simulink model "My_own_6dofblock"  (R2024b)
settings: Solver=VariableStepAuto  StartTime=0.0  StopTime=10.0  RelTol=1e-3
settings Model: Creator=Thetw  LastModifiedBy=Thetw

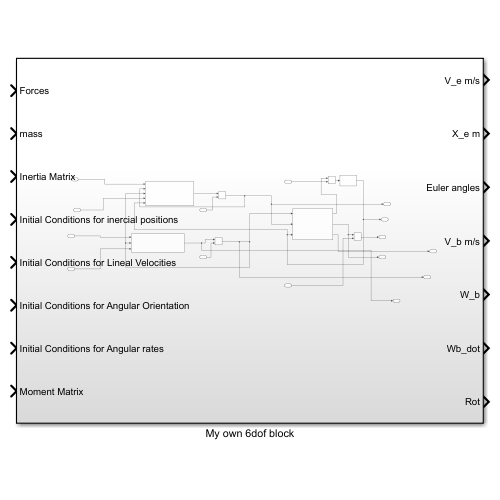
[thumbnail: Simulink's stored preview of the top-level diagram]
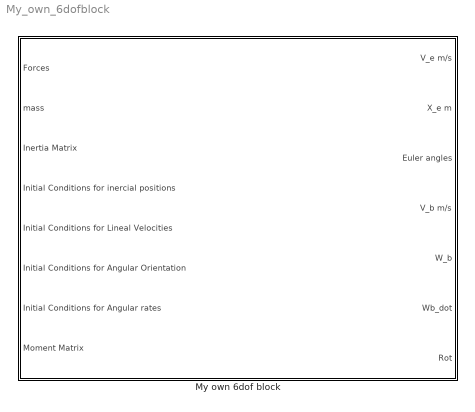
== system My_own_6dofblock ==
  My own 6dof block : Subsystem

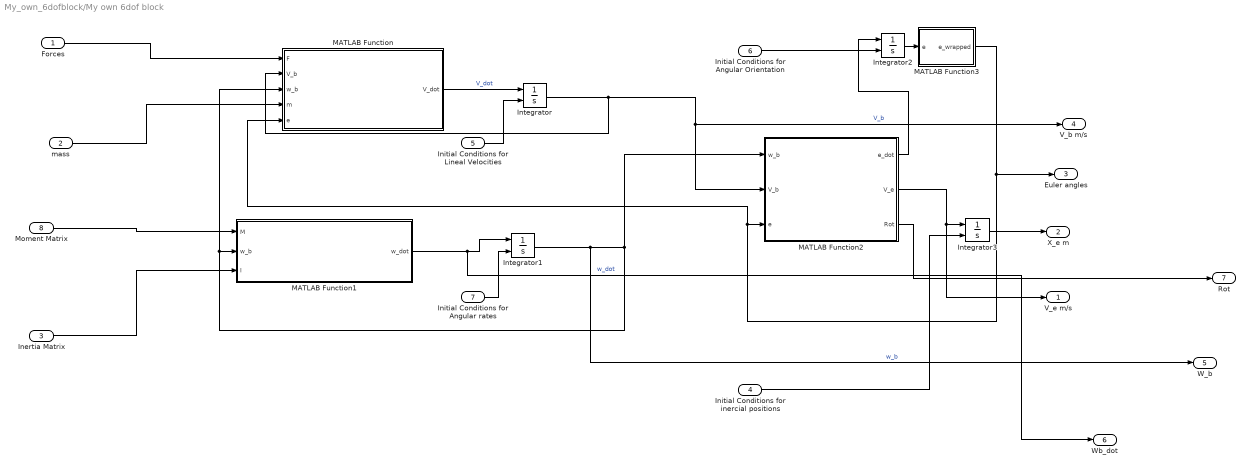
== system My_own_6dofblock/My own 6dof block ==
  Forces : Inport
  mass : Inport  Port=2
  Inertia Matrix : Inport  Port=3
  Initial Conditions for inercial positions : Inport  Port=4
  Initial Conditions for Lineal Velocities : Inport  Port=5
  Initial Conditions for Angular Orientation : Inport  Port=6
  Initial Conditions for Angular rates : Inport  Port=7
  Moment Matrix : Inport  Port=8
  Integrator{,1..3} (4 alike) : Integrator  InitialConditionSource=external
  MATLAB Function : MATLAB Function  TreatAsAtomicUnit=on
  MATLAB Function1 : MATLAB Function  TreatAsAtomicUnit=on
  MATLAB Function2 : MATLAB Function  TreatAsAtomicUnit=on
  MATLAB Function3 : MATLAB Function  TreatAsAtomicUnit=on
  V_e m/s : Outport
  X_e m : Outport  Port=2
  Euler angles : Outport  Port=3
  V_b m/s : Outport  Port=4
  W_b : Outport  Port=5
  Wb_dot : Outport  Port=6
  Rot : Outport  Port=7
  wires:
  Integrator1/1 -> W_b/1, MATLAB Function2/1(w_b), MATLAB Function/3(w_b), MATLAB Function1/2(w_b)  "w_b"
  MATLAB Function/1(V_dot) -> Integrator/1  "V_dot"
  Integrator2/1 -> MATLAB Function3/1(e)
  MATLAB Function2/2(V_e) -> V_e m/s/1, Integrator3/1
  mass/1 -> MATLAB Function/4(m)
  MATLAB Function2/1(e_dot) -> Integrator2/1
  MATLAB Function1/1(w_dot) -> Wb_dot/1, Integrator1/1  "w_dot"
  Integrator3/1 -> X_e m/1
  Integrator/1 -> MATLAB Function/2(V_b), V_b m/s/1, MATLAB Function2/2(V_b)  "V_b"
  Inertia Matrix/1 -> MATLAB Function1/3(I)
  Forces/1 -> MATLAB Function/1(F)
  Moment Matrix/1 -> MATLAB Function1/1(M)
  Initial Conditions for Lineal Velocities/1 -> Integrator/2
  Initial Conditions for Angular rates/1 -> Integrator1/2
  Initial Conditions for inercial positions/1 -> Integrator3/2
  MATLAB Function2/3(Rot) -> Rot/1
  Initial Conditions for Angular Orientation/1 -> Integrator2/2
  MATLAB Function3/1(e_wrapped) -> Euler angles/1, MATLAB Function/5(e), MATLAB Function2/3(e)

== matlab function My_own_6dofblock/My own 6dof block/MATLAB Function ==
  data: F input; V_dot output; V_b input; w_b input; m input; e input
 function V_dot = Traslational_Dynamics(F, V_b, w_b, m, e)

    % Force inputs into a column vector
    F   = F(:);
    V_b = V_b(:);
    w_b = w_b(:);

    % Coriolis effect 
    cross_term = cross(w_b, V_b);


    
    phi = e(1);
    theta = e(2);
    psi = e(3);

    % --- Rotation Matrix ---
    cpsi = cos(psi); spsi = sin(psi);
    cth = cos(theta); sth = sin(theta);
    cphi = cos(phi); sphi = sin(phi);

    R_eb = [ ...
        cth*cpsi,  sphi*sth*cpsi - cphi*spsi,  cphi*sth*cpsi + sphi*spsi;
        cth*spsi,  sphi*sth*spsi + cphi*cpsi,  cphi*sth*spsi - sphi*cpsi;
        -sth,       sphi*cth,                 cphi*cth ];

    Rot = R_eb

    % Traslational Dynamics
    V_dot = (F / m) - cross_term;

  
end

== matlab function My_own_6dofblock/My own 6dof block/MATLAB Function1 ==
  data: M input; w_dot output; w_b input; I input
function w_dot = Rotational_Dynamics(M, w_b, I)

    % Force inputs into a column vector
    M   = M(:);
    w_b = w_b(:);

    % Dot procut for the Inertia term
    Iw_b = I * w_b;

    % Cross product
    cross_term = cross(w_b, Iw_b);

    % Rotational Dynamics op
    w_dot = I \ (M - cross_term);
end

== matlab function My_own_6dofblock/My own 6dof block/MATLAB Function2 ==
  data: w_b input; e_dot output; V_b input; e input; V_e output; Rot output
function [e_dot, V_e, Rot] = Kinematics(w_b, V_b, e)

    % Force inputs into a column vectora
    w_b = w_b(:);
    V_b = V_b(:);
    e   = e(:);

    phi = e(1);
    theta = e(2);
    psi = e(3);

    % --- J Matrix ---
    J_e = [ ...
        1, sin(phi)*tan(theta),  cos(phi)*tan(theta);
        0,      cos(phi),       -sin(phi);
        0, sin(phi)/cos(theta),  cos(phi)/cos(theta) ];

    % Euler Derivation
    e_dot = J_e * w_b;   % → 3x1

    % --- Rotation Matrix ---
    cpsi = cos(psi); spsi = sin(psi);
    cth = cos(theta); sth = sin(theta);
    cphi = cos(phi); sphi = sin(phi);

    R_eb = [ ...
        cth*cpsi,  sphi*sth*cpsi - cphi*spsi,  cphi*sth*cpsi + sphi*spsi;
        cth*spsi,  sphi*sth*spsi + cphi*cpsi,  cphi*sth*spsi - sphi*cpsi;
        -sth,       sphi*cth,                 cphi*cth ];

    Rot = R_eb


    
    % Inertial rates
    V_e = R_eb * V_b;   % → 3x1

end

== matlab function My_own_6dofblock/My own 6dof block/MATLAB Function3 ==
  data: e input; e_wrapped output
function e_wrapped = WrapEuler(e)
% Envuelve cada ángulo a (-pi, pi]

    % Aseguramos vector columna
    e = e(:);

    % Envolver elemento a elemento
    e_wrapped = atan2(sin(e), cos(e));
end
